simulink model "podc2012B"  (R2012b)
settings: Solver=ode45  StartTime=0.0  StopTime=5  RelTol=1e-3
libraries: fuzblock x1
settings Model: Creator=Sandra Knezevic  LastModifiedBy=Aldin
settings OptimizationCC: ExpressionDepthLimit=128
settings DebuggingCC: UnderspecifiedInitializationDetection=Simplified  MergeDetectMultiDrivingBlocksExec=error  SolverPrmCheckMsg=none  FrameProcessingCompatibilityMsg=error  StateNameClashWarn=none
settings CodeAppCC: CustomSymbolStrType=$N$R$M_T
settings GRTTargetCC: CodeReplacementLibrary=C89/C90 (ANSI)

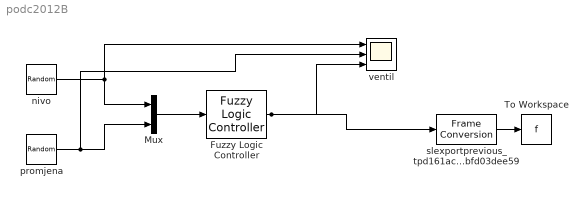
== system podc2012B ==
  Fuzzy Logic Controller : fuzblock/Fuzzy Logic  Controller  FIS=fazzi
  Mux : Mux  Inputs=2
  To Workspace : ToWorkspace  VariableName=f  SampleTime=-1
  nivo : RandomNumber  Mean=-1  SampleTime=0.1
  promjena : RandomNumber  Mean=-0.55  Variance=0.55  SampleTime=0.1
  slexportprevious_tpd161ac58_ee54_435b_bbae_77bfd03dee59 : FrameConversion  OutFrame=Sample-based
  ventil : Scope  NumInputPorts=3
      settings: TimeRange=auto  TickLabels=on  ShowLegends=on  LimitDataPoints=on  MaxDataPoints=5000  SaveToWorkspace=off  SaveName=ScopeData  YMin=-5~-5~-5  YMax=5~5~5  SampleTime=-1  DataFormat=Array
  wires:
  Fuzzy Logic Controller/1 -> ventil/3, slexportprevious_tpd161ac58_ee54_435b_bbae_77bfd03dee59/1
  Mux/1 -> Fuzzy Logic Controller/1
  promjena/1 -> ventil/2, Mux/2
  nivo/1 -> Mux/1, ventil/1
  slexportprevious_tpd161ac58_ee54_435b_bbae_77bfd03dee59/1 -> To Workspace/1
